simulink model "chap04_46"  (R2021a)
settings: Solver=FixedStepDiscrete  StartTime=0.0  StopTime=30  FixedStep=0.001  RelTol=1e-3
undefined symbols (not defined in the file): DiscIntNeverNeededParam
libraries: simulink x4
(part 4 of 4)

== system chap04_46/Subsystem/Subsystem2/Subsystem3/Subsystem ==
  e1 : Inport
  k3 : Inport  Port=2
  k4 : Inport  Port=3
  Add : Sum
  Constant3 : Constant  Value=-1
  Constant4 : Constant  Value=-1
  Discrete-Time Integrator1 : DiscreteIntegrator  SampleTime=-1  ICPrevOutput=DiscIntNeverNeededParam  ICPrevScaledInput=DiscIntNeverNeededParam
  Divide : Product  Inputs=*/
  MATLAB Function : MATLAB Function  TreatAsAtomicUnit=on
  Product3 : Product  Inputs=3
  Product5 : Product  Inputs=3
  z2 : Outport
  wires:
  Constant4/1 -> Product5/1
  Product5/1 -> Add/2
  Discrete-Time Integrator1/1 -> z2/1
  k3/1 -> Product3/3
  k4/1 -> Product5/3
  Divide/1 -> Add/1
  Add/1 -> Discrete-Time Integrator1/1
  Constant3/1 -> Product3/1
  e1/1 -> Product5/2, MATLAB Function/1(u), Product3/2
  MATLAB Function/1(y) -> Divide/2
  Product3/1 -> Divide/1

== system chap04_46/Subsystem/Subsystem2/Subsystem3/Subsystem1 ==
  e1 : Inport
  k1 : Inport  Port=2
  Constant : Constant  Value=-1
  Divide : Product  Inputs=*/
  MATLAB Function : MATLAB Function  TreatAsAtomicUnit=on
  Product : Product  Inputs=3
  Out1 : Outport
  wires:
  e1/1 -> Product/2, MATLAB Function/1(u)
  Divide/1 -> Out1/1
  Constant/1 -> Product/1
  k1/1 -> Product/3
  MATLAB Function/1(y) -> Divide/2
  Product/1 -> Divide/1

== system chap04_46/Subsystem/Subsystem2/Subsystem3/Subsystem2 ==
  e1 : Inport
  Constant1 : Constant  Value=0.2
  Discrete-Time Integrator1 : DiscreteIntegrator  gainval=1  InitialCondition=0.25  SampleTime=-1  ICPrevOutput=DiscIntNeverNeededParam  ICPrevScaledInput=DiscIntNeverNeededParam
  MATLAB Function : MATLAB Function  TreatAsAtomicUnit=on
  Product{,1..3,6} (5 alike) : Product
  Scope1 : Scope
  Sqrt : Sqrt  SaturateOnIntegerOverflow=on
  Square : Math  Operator=square  SaturateOnIntegerOverflow=on
  Subtract2 : Sum  Inputs=+-
  c1 : Constant  Value=0.3
  c2 : Constant  Value=0.3
  c3 : Constant  Value=0.5
  c4 : Constant  Value=0.5
  k1 : Outport
  k2 : Outport  Port=2
  k3 : Outport  Port=3
  k4 : Outport  Port=4
  wires:
  c2/1 -> Product/1
  Product/1 -> k2/1
  c3/1 -> Product1/1
  Product1/1 -> k3/1
  c4/1 -> Product2/1
  Product2/1 -> k4/1
  c1/1 -> Product3/1
  Product3/1 -> k1/1
  Sqrt/1 -> Product3/2
  Square/1 -> Product2/2
  e1/1 -> MATLAB Function/1(u)
  Product6/1 -> Subtract2/2
  MATLAB Function/1(y) -> Subtract2/1
  Subtract2/1 -> Discrete-Time Integrator1/1
  Constant1/1 -> Product6/1
  Discrete-Time Integrator1/1 -> Product6/2, Sqrt/1, Product/2, Square/1, Product1/2, Scope1/1

== system chap04_46/Subsystem/Subsystem2/Subsystem3/Subsystem3 ==
  e1 : Inport
  k2 : Inport  Port=2
  Constant2 : Constant  Value=-1
  Product2 : Product  Inputs=3
  Out1 : Outport
  wires:
  Product2/1 -> Out1/1
  e1/1 -> Product2/2
  k2/1 -> Product2/3
  Constant2/1 -> Product2/1

== system chap04_46/Subsystem/Subsystem2/Subsystem4/Subsystem ==
  zt3 : Inport
  Constant4 : Constant  Value=0
  Discrete-Time Integrator : DiscreteIntegrator  SampleTime=-1  UpperSaturationLimit=100  LowerSaturationLimit=-100  ICPrevOutput=DiscIntNeverNeededParam  ICPrevScaledInput=DiscIntNeverNeededParam
  Logical Operator : Logic  AllPortsSameDT=off  OutDataTypeStr=boolean
  MATLAB Function : MATLAB Function  TreatAsAtomicUnit=on
  Relational Operator : RelationalOperator  Operator===  OutDataTypeStr=boolean  RndMeth=Simplest
  Saturation : Saturate  UpperLimit=5  LowerLimit=-5
  Sign : Signum
  Sign1 : Signum
  Switch : Switch  Criteria=u2 > Threshold
  Out1 : Outport
  wires:
  MATLAB Function/1(y) -> Logical Operator/1
  Relational Operator/1 -> Logical Operator/2
  Constant4/1 -> Switch/1
  Sign1/1 -> Relational Operator/1
  zt3/1 -> Sign1/1, Switch/3
  Saturation/1 -> Out1/1, MATLAB Function/2(u2)
  Discrete-Time Integrator/1 -> Saturation/1, MATLAB Function/1(u1), Sign/1
  Sign/1 -> Relational Operator/2
  Logical Operator/1 -> Switch/2
  Switch/1 -> Discrete-Time Integrator/1

== system chap04_46/Subsystem/Subsystem2/Subsystem7/Subsystem ==
  zt3 : Inport
  Constant4 : Constant  Value=0
  Discrete-Time Integrator : DiscreteIntegrator  SampleTime=-1  UpperSaturationLimit=100  LowerSaturationLimit=-100  ICPrevOutput=DiscIntNeverNeededParam  ICPrevScaledInput=DiscIntNeverNeededParam
  Logical Operator : Logic  AllPortsSameDT=off  OutDataTypeStr=boolean
  MATLAB Function : MATLAB Function  TreatAsAtomicUnit=on
  Relational Operator : RelationalOperator  Operator===  OutDataTypeStr=boolean  RndMeth=Simplest
  Saturation : Saturate  UpperLimit=5  LowerLimit=-5
  Sign : Signum
  Sign1 : Signum
  Switch : Switch  Criteria=u2 > Threshold
  Out1 : Outport
  wires:
  Switch/1 -> Discrete-Time Integrator/1
  Logical Operator/1 -> Switch/2
  Sign/1 -> Relational Operator/2
  Discrete-Time Integrator/1 -> Sign/1, MATLAB Function/1(u1), Saturation/1
  Saturation/1 -> MATLAB Function/2(u2), Out1/1
  zt3/1 -> Switch/3, Sign1/1
  Sign1/1 -> Relational Operator/1
  Constant4/1 -> Switch/1
  Relational Operator/1 -> Logical Operator/2
  MATLAB Function/1(y) -> Logical Operator/1

== system chap04_46/Subsystem/Subsystem2/Subsystem8/Subsystem ==
  zt3 : Inport
  Constant4 : Constant  Value=0
  Discrete-Time Integrator : DiscreteIntegrator  SampleTime=-1  UpperSaturationLimit=100  LowerSaturationLimit=-100  ICPrevOutput=DiscIntNeverNeededParam  ICPrevScaledInput=DiscIntNeverNeededParam
  Logical Operator : Logic  AllPortsSameDT=off  OutDataTypeStr=boolean
  MATLAB Function : MATLAB Function  TreatAsAtomicUnit=on
  Relational Operator : RelationalOperator  Operator===  OutDataTypeStr=boolean  RndMeth=Simplest
  Saturation : Saturate  UpperLimit=5  LowerLimit=-5
  Sign : Signum
  Sign1 : Signum
  Switch : Switch  Criteria=u2 > Threshold
  Out1 : Outport
  wires:
  MATLAB Function/1(y) -> Logical Operator/1
  Relational Operator/1 -> Logical Operator/2
  Constant4/1 -> Switch/1
  Sign1/1 -> Relational Operator/1
  zt3/1 -> Sign1/1, Switch/3
  Saturation/1 -> Out1/1, MATLAB Function/2(u2)
  Discrete-Time Integrator/1 -> Saturation/1, MATLAB Function/1(u1), Sign/1
  Sign/1 -> Relational Operator/2
  Logical Operator/1 -> Switch/2
  Switch/1 -> Discrete-Time Integrator/1

== system chap04_46/Subsystem/Subsystem3/Subsystem3/Subsystem ==
  e1 : Inport
  k3 : Inport  Port=2
  k4 : Inport  Port=3
  Add : Sum
  Constant3 : Constant  Value=-1
  Constant4 : Constant  Value=-1
  Discrete-Time Integrator1 : DiscreteIntegrator  SampleTime=-1  ICPrevOutput=DiscIntNeverNeededParam  ICPrevScaledInput=DiscIntNeverNeededParam
  Divide : Product  Inputs=*/
  MATLAB Function : MATLAB Function  TreatAsAtomicUnit=on
  Product3 : Product  Inputs=3
  Product5 : Product  Inputs=3
  z2 : Outport
  wires:
  Constant4/1 -> Product5/1
  Product5/1 -> Add/2
  Discrete-Time Integrator1/1 -> z2/1
  k3/1 -> Product3/3
  k4/1 -> Product5/3
  Divide/1 -> Add/1
  Add/1 -> Discrete-Time Integrator1/1
  Constant3/1 -> Product3/1
  e1/1 -> Product5/2, MATLAB Function/1(u), Product3/2
  MATLAB Function/1(y) -> Divide/2
  Product3/1 -> Divide/1

== system chap04_46/Subsystem/Subsystem3/Subsystem3/Subsystem1 ==
  e1 : Inport
  k1 : Inport  Port=2
  Constant : Constant  Value=-1
  Divide : Product  Inputs=*/
  MATLAB Function : MATLAB Function  TreatAsAtomicUnit=on
  Product : Product  Inputs=3
  Out1 : Outport
  wires:
  e1/1 -> Product/2, MATLAB Function/1(u)
  Divide/1 -> Out1/1
  Constant/1 -> Product/1
  k1/1 -> Product/3
  MATLAB Function/1(y) -> Divide/2
  Product/1 -> Divide/1

== system chap04_46/Subsystem/Subsystem3/Subsystem3/Subsystem2 ==
  e1 : Inport
  Constant1 : Constant  Value=0.2
  Discrete-Time Integrator1 : DiscreteIntegrator  gainval=1  InitialCondition=0.25  SampleTime=-1  ICPrevOutput=DiscIntNeverNeededParam  ICPrevScaledInput=DiscIntNeverNeededParam
  MATLAB Function : MATLAB Function  TreatAsAtomicUnit=on
  Product{,1..3,6} (5 alike) : Product
  Scope1 : Scope
  Sqrt : Sqrt  SaturateOnIntegerOverflow=on
  Square : Math  Operator=square  SaturateOnIntegerOverflow=on
  Subtract2 : Sum  Inputs=+-
  c1 : Constant  Value=0.3
  c2 : Constant  Value=0.3
  c3 : Constant  Value=0.5
  c4 : Constant  Value=0.5
  k1 : Outport
  k2 : Outport  Port=2
  k3 : Outport  Port=3
  k4 : Outport  Port=4
  wires:
  c2/1 -> Product/1
  Product/1 -> k2/1
  c3/1 -> Product1/1
  Product1/1 -> k3/1
  c4/1 -> Product2/1
  Product2/1 -> k4/1
  c1/1 -> Product3/1
  Product3/1 -> k1/1
  Sqrt/1 -> Product3/2
  Square/1 -> Product2/2
  e1/1 -> MATLAB Function/1(u)
  Product6/1 -> Subtract2/2
  MATLAB Function/1(y) -> Subtract2/1
  Subtract2/1 -> Discrete-Time Integrator1/1
  Constant1/1 -> Product6/1
  Discrete-Time Integrator1/1 -> Product6/2, Sqrt/1, Product/2, Square/1, Product1/2, Scope1/1

== system chap04_46/Subsystem/Subsystem3/Subsystem3/Subsystem3 ==
  e1 : Inport
  k2 : Inport  Port=2
  Constant2 : Constant  Value=-1
  Product2 : Product  Inputs=3
  Out1 : Outport
  wires:
  Product2/1 -> Out1/1
  e1/1 -> Product2/2
  k2/1 -> Product2/3
  Constant2/1 -> Product2/1

== system chap04_46/Subsystem/Subsystem3/Subsystem4/Subsystem ==
  zt3 : Inport
  Constant4 : Constant  Value=0
  Discrete-Time Integrator : DiscreteIntegrator  SampleTime=-1  UpperSaturationLimit=100  LowerSaturationLimit=-100  ICPrevOutput=DiscIntNeverNeededParam  ICPrevScaledInput=DiscIntNeverNeededParam
  Logical Operator : Logic  AllPortsSameDT=off  OutDataTypeStr=boolean
  MATLAB Function : MATLAB Function  TreatAsAtomicUnit=on
  Relational Operator : RelationalOperator  Operator===  OutDataTypeStr=boolean  RndMeth=Simplest
  Saturation : Saturate  UpperLimit=5  LowerLimit=-5
  Sign : Signum
  Sign1 : Signum
  Switch : Switch  Criteria=u2 > Threshold
  Out1 : Outport
  wires:
  MATLAB Function/1(y) -> Logical Operator/1
  Relational Operator/1 -> Logical Operator/2
  Constant4/1 -> Switch/1
  Sign1/1 -> Relational Operator/1
  zt3/1 -> Sign1/1, Switch/3
  Saturation/1 -> Out1/1, MATLAB Function/2(u2)
  Discrete-Time Integrator/1 -> Saturation/1, MATLAB Function/1(u1), Sign/1
  Sign/1 -> Relational Operator/2
  Logical Operator/1 -> Switch/2
  Switch/1 -> Discrete-Time Integrator/1

== system chap04_46/Subsystem/Subsystem3/Subsystem7/Subsystem ==
  zt3 : Inport
  Constant4 : Constant  Value=0
  Discrete-Time Integrator : DiscreteIntegrator  SampleTime=-1  UpperSaturationLimit=100  LowerSaturationLimit=-100  ICPrevOutput=DiscIntNeverNeededParam  ICPrevScaledInput=DiscIntNeverNeededParam
  Logical Operator : Logic  AllPortsSameDT=off  OutDataTypeStr=boolean
  MATLAB Function : MATLAB Function  TreatAsAtomicUnit=on
  Relational Operator : RelationalOperator  Operator===  OutDataTypeStr=boolean  RndMeth=Simplest
  Saturation : Saturate  UpperLimit=5  LowerLimit=-5
  Sign : Signum
  Sign1 : Signum
  Switch : Switch  Criteria=u2 > Threshold
  Out1 : Outport
  wires:
  Switch/1 -> Discrete-Time Integrator/1
  Logical Operator/1 -> Switch/2
  Sign/1 -> Relational Operator/2
  Discrete-Time Integrator/1 -> Sign/1, MATLAB Function/1(u1), Saturation/1
  Saturation/1 -> MATLAB Function/2(u2), Out1/1
  zt3/1 -> Switch/3, Sign1/1
  Sign1/1 -> Relational Operator/1
  Constant4/1 -> Switch/1
  Relational Operator/1 -> Logical Operator/2
  MATLAB Function/1(y) -> Logical Operator/1

== system chap04_46/Subsystem/Subsystem3/Subsystem8/Subsystem ==
  zt3 : Inport
  Constant4 : Constant  Value=0
  Discrete-Time Integrator : DiscreteIntegrator  SampleTime=-1  UpperSaturationLimit=100  LowerSaturationLimit=-100  ICPrevOutput=DiscIntNeverNeededParam  ICPrevScaledInput=DiscIntNeverNeededParam
  Logical Operator : Logic  AllPortsSameDT=off  OutDataTypeStr=boolean
  MATLAB Function : MATLAB Function  TreatAsAtomicUnit=on
  Relational Operator : RelationalOperator  Operator===  OutDataTypeStr=boolean  RndMeth=Simplest
  Saturation : Saturate  UpperLimit=5  LowerLimit=-5
  Sign : Signum
  Sign1 : Signum
  Switch : Switch  Criteria=u2 > Threshold
  Out1 : Outport
  wires:
  MATLAB Function/1(y) -> Logical Operator/1
  Relational Operator/1 -> Logical Operator/2
  Constant4/1 -> Switch/1
  Sign1/1 -> Relational Operator/1
  zt3/1 -> Sign1/1, Switch/3
  Saturation/1 -> Out1/1, MATLAB Function/2(u2)
  Discrete-Time Integrator/1 -> Saturation/1, MATLAB Function/1(u1), Sign/1
  Sign/1 -> Relational Operator/2
  Logical Operator/1 -> Switch/2
  Switch/1 -> Discrete-Time Integrator/1

== system chap04_46/Subsystem/Subsystem4/Subsystem3/Subsystem ==
  e1 : Inport
  k3 : Inport  Port=2
  k4 : Inport  Port=3
  Add : Sum
  Constant3 : Constant  Value=-1
  Constant4 : Constant  Value=-1
  Discrete-Time Integrator1 : DiscreteIntegrator  SampleTime=-1  ICPrevOutput=DiscIntNeverNeededParam  ICPrevScaledInput=DiscIntNeverNeededParam
  Divide : Product  Inputs=*/
  MATLAB Function : MATLAB Function  TreatAsAtomicUnit=on
  Product3 : Product  Inputs=3
  Product5 : Product  Inputs=3
  z2 : Outport
  wires:
  Constant4/1 -> Product5/1
  Product5/1 -> Add/2
  Discrete-Time Integrator1/1 -> z2/1
  k3/1 -> Product3/3
  k4/1 -> Product5/3
  Divide/1 -> Add/1
  Add/1 -> Discrete-Time Integrator1/1
  Constant3/1 -> Product3/1
  e1/1 -> Product5/2, MATLAB Function/1(u), Product3/2
  MATLAB Function/1(y) -> Divide/2
  Product3/1 -> Divide/1

== system chap04_46/Subsystem/Subsystem4/Subsystem3/Subsystem1 ==
  e1 : Inport
  k1 : Inport  Port=2
  Constant : Constant  Value=-1
  Divide : Product  Inputs=*/
  MATLAB Function : MATLAB Function  TreatAsAtomicUnit=on
  Product : Product  Inputs=3
  Out1 : Outport
  wires:
  e1/1 -> Product/2, MATLAB Function/1(u)
  Divide/1 -> Out1/1
  Constant/1 -> Product/1
  k1/1 -> Product/3
  MATLAB Function/1(y) -> Divide/2
  Product/1 -> Divide/1

== system chap04_46/Subsystem/Subsystem4/Subsystem3/Subsystem2 ==
  e1 : Inport
  Constant1 : Constant  Value=0.2
  Discrete-Time Integrator1 : DiscreteIntegrator  gainval=1  InitialCondition=0.25  SampleTime=-1  ICPrevOutput=DiscIntNeverNeededParam  ICPrevScaledInput=DiscIntNeverNeededParam
  MATLAB Function : MATLAB Function  TreatAsAtomicUnit=on
  Product{,1..3,6} (5 alike) : Product
  Scope1 : Scope
  Sqrt : Sqrt  SaturateOnIntegerOverflow=on
  Square : Math  Operator=square  SaturateOnIntegerOverflow=on
  Subtract2 : Sum  Inputs=+-
  c1 : Constant  Value=0.3
  c2 : Constant  Value=0.3
  c3 : Constant  Value=0.5
  c4 : Constant  Value=0.5
  k1 : Outport
  k2 : Outport  Port=2
  k3 : Outport  Port=3
  k4 : Outport  Port=4
  wires:
  c2/1 -> Product/1
  Product/1 -> k2/1
  c3/1 -> Product1/1
  Product1/1 -> k3/1
  c4/1 -> Product2/1
  Product2/1 -> k4/1
  c1/1 -> Product3/1
  Product3/1 -> k1/1
  Sqrt/1 -> Product3/2
  Square/1 -> Product2/2
  e1/1 -> MATLAB Function/1(u)
  Product6/1 -> Subtract2/2
  MATLAB Function/1(y) -> Subtract2/1
  Subtract2/1 -> Discrete-Time Integrator1/1
  Constant1/1 -> Product6/1
  Discrete-Time Integrator1/1 -> Product6/2, Sqrt/1, Product/2, Square/1, Product1/2, Scope1/1

== system chap04_46/Subsystem/Subsystem4/Subsystem3/Subsystem3 ==
  e1 : Inport
  k2 : Inport  Port=2
  Constant2 : Constant  Value=-1
  Product2 : Product  Inputs=3
  Out1 : Outport
  wires:
  Product2/1 -> Out1/1
  e1/1 -> Product2/2
  k2/1 -> Product2/3
  Constant2/1 -> Product2/1

== system chap04_46/Subsystem/Subsystem4/Subsystem4/Subsystem ==
  zt3 : Inport
  Constant4 : Constant  Value=0
  Discrete-Time Integrator : DiscreteIntegrator  SampleTime=-1  UpperSaturationLimit=100  LowerSaturationLimit=-100  ICPrevOutput=DiscIntNeverNeededParam  ICPrevScaledInput=DiscIntNeverNeededParam
  Logical Operator : Logic  AllPortsSameDT=off  OutDataTypeStr=boolean
  MATLAB Function : MATLAB Function  TreatAsAtomicUnit=on
  Relational Operator : RelationalOperator  Operator===  OutDataTypeStr=boolean  RndMeth=Simplest
  Saturation : Saturate  UpperLimit=5  LowerLimit=-5
  Sign : Signum
  Sign1 : Signum
  Switch : Switch  Criteria=u2 > Threshold
  Out1 : Outport
  wires:
  MATLAB Function/1(y) -> Logical Operator/1
  Relational Operator/1 -> Logical Operator/2
  Constant4/1 -> Switch/1
  Sign1/1 -> Relational Operator/1
  zt3/1 -> Sign1/1, Switch/3
  Saturation/1 -> Out1/1, MATLAB Function/2(u2)
  Discrete-Time Integrator/1 -> Saturation/1, MATLAB Function/1(u1), Sign/1
  Sign/1 -> Relational Operator/2
  Logical Operator/1 -> Switch/2
  Switch/1 -> Discrete-Time Integrator/1

== system chap04_46/Subsystem/Subsystem4/Subsystem7/Subsystem ==
  zt3 : Inport
  Constant4 : Constant  Value=0
  Discrete-Time Integrator : DiscreteIntegrator  SampleTime=-1  UpperSaturationLimit=100  LowerSaturationLimit=-100  ICPrevOutput=DiscIntNeverNeededParam  ICPrevScaledInput=DiscIntNeverNeededParam
  Logical Operator : Logic  AllPortsSameDT=off  OutDataTypeStr=boolean
  MATLAB Function : MATLAB Function  TreatAsAtomicUnit=on
  Relational Operator : RelationalOperator  Operator===  OutDataTypeStr=boolean  RndMeth=Simplest
  Saturation : Saturate  UpperLimit=5  LowerLimit=-5
  Sign : Signum
  Sign1 : Signum
  Switch : Switch  Criteria=u2 > Threshold
  Out1 : Outport
  wires:
  Switch/1 -> Discrete-Time Integrator/1
  Logical Operator/1 -> Switch/2
  Sign/1 -> Relational Operator/2
  Discrete-Time Integrator/1 -> Sign/1, MATLAB Function/1(u1), Saturation/1
  Saturation/1 -> MATLAB Function/2(u2), Out1/1
  zt3/1 -> Switch/3, Sign1/1
  Sign1/1 -> Relational Operator/1
  Constant4/1 -> Switch/1
  Relational Operator/1 -> Logical Operator/2
  MATLAB Function/1(y) -> Logical Operator/1

== system chap04_46/Subsystem/Subsystem4/Subsystem8/Subsystem ==
  zt3 : Inport
  Constant4 : Constant  Value=0
  Discrete-Time Integrator : DiscreteIntegrator  SampleTime=-1  UpperSaturationLimit=100  LowerSaturationLimit=-100  ICPrevOutput=DiscIntNeverNeededParam  ICPrevScaledInput=DiscIntNeverNeededParam
  Logical Operator : Logic  AllPortsSameDT=off  OutDataTypeStr=boolean
  MATLAB Function : MATLAB Function  TreatAsAtomicUnit=on
  Relational Operator : RelationalOperator  Operator===  OutDataTypeStr=boolean  RndMeth=Simplest
  Saturation : Saturate  UpperLimit=5  LowerLimit=-5
  Sign : Signum
  Sign1 : Signum
  Switch : Switch  Criteria=u2 > Threshold
  Out1 : Outport
  wires:
  MATLAB Function/1(y) -> Logical Operator/1
  Relational Operator/1 -> Logical Operator/2
  Constant4/1 -> Switch/1
  Sign1/1 -> Relational Operator/1
  zt3/1 -> Sign1/1, Switch/3
  Saturation/1 -> Out1/1, MATLAB Function/2(u2)
  Discrete-Time Integrator/1 -> Saturation/1, MATLAB Function/1(u1), Sign/1
  Sign/1 -> Relational Operator/2
  Logical Operator/1 -> Switch/2
  Switch/1 -> Discrete-Time Integrator/1

== system chap04_46/Subsystem/Subsystem5/Subsystem3/Subsystem ==
  e1 : Inport
  k3 : Inport  Port=2
  k4 : Inport  Port=3
  Add : Sum
  Constant3 : Constant  Value=-1
  Constant4 : Constant  Value=-1
  Discrete-Time Integrator1 : DiscreteIntegrator  SampleTime=-1  ICPrevOutput=DiscIntNeverNeededParam  ICPrevScaledInput=DiscIntNeverNeededParam
  Divide : Product  Inputs=*/
  MATLAB Function : MATLAB Function  TreatAsAtomicUnit=on
  Product3 : Product  Inputs=3
  Product5 : Product  Inputs=3
  z2 : Outport
  wires:
  Constant4/1 -> Product5/1
  Product5/1 -> Add/2
  Discrete-Time Integrator1/1 -> z2/1
  k3/1 -> Product3/3
  k4/1 -> Product5/3
  Divide/1 -> Add/1
  Add/1 -> Discrete-Time Integrator1/1
  Constant3/1 -> Product3/1
  e1/1 -> Product5/2, MATLAB Function/1(u), Product3/2
  MATLAB Function/1(y) -> Divide/2
  Product3/1 -> Divide/1

== system chap04_46/Subsystem/Subsystem5/Subsystem3/Subsystem1 ==
  e1 : Inport
  k1 : Inport  Port=2
  Constant : Constant  Value=-1
  Divide : Product  Inputs=*/
  MATLAB Function : MATLAB Function  TreatAsAtomicUnit=on
  Product : Product  Inputs=3
  Out1 : Outport
  wires:
  e1/1 -> Product/2, MATLAB Function/1(u)
  Divide/1 -> Out1/1
  Constant/1 -> Product/1
  k1/1 -> Product/3
  MATLAB Function/1(y) -> Divide/2
  Product/1 -> Divide/1

== system chap04_46/Subsystem/Subsystem5/Subsystem3/Subsystem2 ==
  e1 : Inport
  Constant1 : Constant  Value=0.2
  Discrete-Time Integrator1 : DiscreteIntegrator  gainval=1  InitialCondition=0.25  SampleTime=-1  ICPrevOutput=DiscIntNeverNeededParam  ICPrevScaledInput=DiscIntNeverNeededParam
  MATLAB Function : MATLAB Function  TreatAsAtomicUnit=on
  Product{,1..3,6} (5 alike) : Product
  Scope1 : Scope
  Sqrt : Sqrt  SaturateOnIntegerOverflow=on
  Square : Math  Operator=square  SaturateOnIntegerOverflow=on
  Subtract2 : Sum  Inputs=+-
  c1 : Constant  Value=0.3
  c2 : Constant  Value=0.3
  c3 : Constant  Value=0.5
  c4 : Constant  Value=0.5
  k1 : Outport
  k2 : Outport  Port=2
  k3 : Outport  Port=3
  k4 : Outport  Port=4
  wires:
  c2/1 -> Product/1
  Product/1 -> k2/1
  c3/1 -> Product1/1
  Product1/1 -> k3/1
  c4/1 -> Product2/1
  Product2/1 -> k4/1
  c1/1 -> Product3/1
  Product3/1 -> k1/1
  Sqrt/1 -> Product3/2
  Square/1 -> Product2/2
  e1/1 -> MATLAB Function/1(u)
  Product6/1 -> Subtract2/2
  MATLAB Function/1(y) -> Subtract2/1
  Subtract2/1 -> Discrete-Time Integrator1/1
  Constant1/1 -> Product6/1
  Discrete-Time Integrator1/1 -> Product6/2, Sqrt/1, Product/2, Square/1, Product1/2, Scope1/1

== system chap04_46/Subsystem/Subsystem5/Subsystem3/Subsystem3 ==
  e1 : Inport
  k2 : Inport  Port=2
  Constant2 : Constant  Value=-1
  Product2 : Product  Inputs=3
  Out1 : Outport
  wires:
  Product2/1 -> Out1/1
  e1/1 -> Product2/2
  k2/1 -> Product2/3
  Constant2/1 -> Product2/1

== system chap04_46/Subsystem/Subsystem5/Subsystem4/Subsystem ==
  zt3 : Inport
  Constant4 : Constant  Value=0
  Discrete-Time Integrator : DiscreteIntegrator  SampleTime=-1  UpperSaturationLimit=100  LowerSaturationLimit=-100  ICPrevOutput=DiscIntNeverNeededParam  ICPrevScaledInput=DiscIntNeverNeededParam
  Logical Operator : Logic  AllPortsSameDT=off  OutDataTypeStr=boolean
  MATLAB Function : MATLAB Function  TreatAsAtomicUnit=on
  Relational Operator : RelationalOperator  Operator===  OutDataTypeStr=boolean  RndMeth=Simplest
  Saturation : Saturate  UpperLimit=5  LowerLimit=-5
  Sign : Signum
  Sign1 : Signum
  Switch : Switch  Criteria=u2 > Threshold
  Out1 : Outport
  wires:
  MATLAB Function/1(y) -> Logical Operator/1
  Relational Operator/1 -> Logical Operator/2
  Constant4/1 -> Switch/1
  Sign1/1 -> Relational Operator/1
  zt3/1 -> Sign1/1, Switch/3
  Saturation/1 -> Out1/1, MATLAB Function/2(u2)
  Discrete-Time Integrator/1 -> Saturation/1, MATLAB Function/1(u1), Sign/1
  Sign/1 -> Relational Operator/2
  Logical Operator/1 -> Switch/2
  Switch/1 -> Discrete-Time Integrator/1

== system chap04_46/Subsystem/Subsystem5/Subsystem7/Subsystem ==
  zt3 : Inport
  Constant4 : Constant  Value=0
  Discrete-Time Integrator : DiscreteIntegrator  SampleTime=-1  UpperSaturationLimit=100  LowerSaturationLimit=-100  ICPrevOutput=DiscIntNeverNeededParam  ICPrevScaledInput=DiscIntNeverNeededParam
  Logical Operator : Logic  AllPortsSameDT=off  OutDataTypeStr=boolean
  MATLAB Function : MATLAB Function  TreatAsAtomicUnit=on
  Relational Operator : RelationalOperator  Operator===  OutDataTypeStr=boolean  RndMeth=Simplest
  Saturation : Saturate  UpperLimit=5  LowerLimit=-5
  Sign : Signum
  Sign1 : Signum
  Switch : Switch  Criteria=u2 > Threshold
  Out1 : Outport
  wires:
  Switch/1 -> Discrete-Time Integrator/1
  Logical Operator/1 -> Switch/2
  Sign/1 -> Relational Operator/2
  Discrete-Time Integrator/1 -> Sign/1, MATLAB Function/1(u1), Saturation/1
  Saturation/1 -> MATLAB Function/2(u2), Out1/1
  zt3/1 -> Switch/3, Sign1/1
  Sign1/1 -> Relational Operator/1
  Constant4/1 -> Switch/1
  Relational Operator/1 -> Logical Operator/2
  MATLAB Function/1(y) -> Logical Operator/1

== system chap04_46/Subsystem/Subsystem5/Subsystem8/Subsystem ==
  zt3 : Inport
  Constant4 : Constant  Value=0
  Discrete-Time Integrator : DiscreteIntegrator  SampleTime=-1  UpperSaturationLimit=100  LowerSaturationLimit=-100  ICPrevOutput=DiscIntNeverNeededParam  ICPrevScaledInput=DiscIntNeverNeededParam
  Logical Operator : Logic  AllPortsSameDT=off  OutDataTypeStr=boolean
  MATLAB Function : MATLAB Function  TreatAsAtomicUnit=on
  Relational Operator : RelationalOperator  Operator===  OutDataTypeStr=boolean  RndMeth=Simplest
  Saturation : Saturate  UpperLimit=5  LowerLimit=-5
  Sign : Signum
  Sign1 : Signum
  Switch : Switch  Criteria=u2 > Threshold
  Out1 : Outport
  wires:
  MATLAB Function/1(y) -> Logical Operator/1
  Relational Operator/1 -> Logical Operator/2
  Constant4/1 -> Switch/1
  Sign1/1 -> Relational Operator/1
  zt3/1 -> Sign1/1, Switch/3
  Saturation/1 -> Out1/1, MATLAB Function/2(u2)
  Discrete-Time Integrator/1 -> Saturation/1, MATLAB Function/1(u1), Sign/1
  Sign/1 -> Relational Operator/2
  Logical Operator/1 -> Switch/2
  Switch/1 -> Discrete-Time Integrator/1

== matlab function chap04_46/Subsystem/Subsystem/Subsystem4/Subsystem/MATLAB Function ==
  data: u1 input; y output; u2 input
function y = fcn(u1,u2)


if (u1==u2)
    y = 0;
else
    y = 1;
end

== matlab function chap04_46/Subsystem/Subsystem5/Subsystem12/MATLAB Function ==
  data: u input; y output
function y = fcn(u)

y = norm(u);

== matlab function chap04_46/Subsystem/Subsystem5/Subsystem4/Subsystem/MATLAB Function ==
  data: u1 input; y output; u2 input
function y = fcn(u1,u2)


if (u1==u2)
    y = 0;
else
    y = 1;
end

== matlab function chap04_46/Subsystem/Subsystem5/Subsystem7/Subsystem/MATLAB Function ==
  data: u1 input; y output; u2 input
function y = fcn(u1,u2)


if (u1==u2)
    y = 0;
else
    y = 1;
end

== matlab function chap04_46/Subsystem/Subsystem5/Subsystem8/Subsystem/MATLAB Function ==
  data: u1 input; y output; u2 input
function y = fcn(u1,u2)


if (u1==u2)
    y = 0;
else
    y = 1;
end

== matlab function chap04_46/Subsystem/Subsystem5/Subsystem12/MATLAB Function3 ==
  data: u input; y output
function y = fcn(u)

y = norm(u);

== matlab function chap04_46/Subsystem/Subsystem3/Subsystem12/MATLAB Function ==
  data: u input; y output
function y = fcn(u)

y = norm(u);

== matlab function chap04_46/Subsystem/Subsystem3/Subsystem12/MATLAB Function3 ==
  data: u input; y output
function y = fcn(u)

y = norm(u);

== matlab function chap04_46/Subsystem/Subsystem2/Subsystem7/Subsystem/MATLAB Function ==
  data: u1 input; y output; u2 input
function y = fcn(u1,u2)


if (u1==u2)
    y = 0;
else
    y = 1;
end

== matlab function chap04_46/Subsystem/Subsystem3/Subsystem4/Subsystem/MATLAB Function ==
  data: u1 input; y output; u2 input
function y = fcn(u1,u2)


if (u1==u2)
    y = 0;
else
    y = 1;
end

== matlab function chap04_46/Subsystem/Subsystem3/Subsystem7/Subsystem/MATLAB Function ==
  data: u1 input; y output; u2 input
function y = fcn(u1,u2)


if (u1==u2)
    y = 0;
else
    y = 1;
end

== matlab function chap04_46/Subsystem/Subsystem4/Subsystem4/Subsystem/MATLAB Function ==
  data: u1 input; y output; u2 input
function y = fcn(u1,u2)


if (u1==u2)
    y = 0;
else
    y = 1;
end

== matlab function chap04_46/Subsystem/Subsystem4/Subsystem7/Subsystem/MATLAB Function ==
  data: u1 input; y output; u2 input
function y = fcn(u1,u2)


if (u1==u2)
    y = 0;
else
    y = 1;
end

== matlab function chap04_46/Subsystem/Subsystem4/Subsystem8/Subsystem/MATLAB Function ==
  data: u1 input; y output; u2 input
function y = fcn(u1,u2)


if (u1==u2)
    y = 0;
else
    y = 1;
end

== matlab function chap04_46/Subsystem/Subsystem3/Subsystem8/Subsystem/MATLAB Function ==
  data: u1 input; y output; u2 input
function y = fcn(u1,u2)


if (u1==u2)
    y = 0;
else
    y = 1;
end

== matlab function chap04_46/Subsystem/Subsystem1/Subsystem12/MATLAB Function ==
  data: u input; y output
function y = fcn(u)

y = norm(u);

== matlab function chap04_46/Subsystem/Subsystem1/Subsystem12/MATLAB Function3 ==
  data: u input; y output
function y = fcn(u)

y = norm(u);

== matlab function chap04_46/Subsystem/Subsystem4/Subsystem12/MATLAB Function ==
  data: u input; y output
function y = fcn(u)

y = norm(u);

== matlab function chap04_46/Subsystem/Subsystem4/Subsystem12/MATLAB Function3 ==
  data: u input; y output
function y = fcn(u)

y = norm(u);

== matlab function chap04_46/Subsystem/Subsystem2/Subsystem3/Subsystem2/MATLAB Function ==
  data: u input; y output
function y = fcn(u)

y = norm(u);

== matlab function chap04_46/Subsystem/Subsystem2/Subsystem8/Subsystem/MATLAB Function ==
  data: u1 input; y output; u2 input
function y = fcn(u1,u2)


if (u1==u2)
    y = 0;
else
    y = 1;
end

== matlab function chap04_46/Subsystem/Subsystem5/Subsystem3/Subsystem2/MATLAB Function ==
  data: u input; y output
function y = fcn(u)

y = norm(u);

== matlab function chap04_46/Subsystem/Subsystem3/Subsystem3/Subsystem2/MATLAB Function ==
  data: u input; y output
function y = fcn(u)

y = norm(u);

== matlab function chap04_46/Subsystem/Subsystem1/Subsystem3/Subsystem2/MATLAB Function ==
  data: u input; y output
function y = fcn(u)

y = norm(u);

== matlab function chap04_46/Subsystem/Subsystem4/Subsystem3/Subsystem2/MATLAB Function ==
  data: u input; y output
function y = fcn(u)

y = norm(u);

== matlab function chap04_46/Subsystem/Subsystem/Subsystem3/MATLAB Function ==
  data: u input; y output
function y = fcn(u)

y = u;

if y==0
    y=10e-15;
end

== matlab function chap04_46/Subsystem/Subsystem/Subsystem3/MATLAB Function1 ==
  data: u input; y output
function y = fcn(u)

y = u;

if y==0
    y=10e-15;
end

== matlab function chap04_46/Subsystem/Subsystem/Subsystem3/MATLAB Function2 ==
  data: u input; y output
function y = fcn(u)

y = u;

if y==0
    y=10e-15;
end

== matlab function chap04_46/Subsystem/Subsystem/Subsystem3/Subsystem/MATLAB Function ==
  data: u input; y output
function y = fcn(u)

y = norm(u);

== matlab function chap04_46/Subsystem/Subsystem/Subsystem3/Subsystem1/MATLAB Function ==
  data: u input; y output
function y = fcn(u)

y = norm(u)^(1/2);

== matlab function chap04_46/Subsystem/Subsystem/Subsystem3/Subsystem2/MATLAB Function ==
  data: u input; y output
function y = fcn(u)

y = norm(u);

== matlab function chap04_46/Subsystem/Subsystem2/Subsystem3/MATLAB Function ==
  data: u input; y output
function y = fcn(u)

y = u;

if y==0
    y=10e-15;
end

== matlab function chap04_46/Subsystem/Subsystem1/Subsystem4/Subsystem/MATLAB Function ==
  data: u1 input; y output; u2 input
function y = fcn(u1,u2)


if (u1==u2)
    y = 0;
else
    y = 1;
end

== matlab function chap04_46/Subsystem/Subsystem2/Subsystem3/MATLAB Function1 ==
  data: u input; y output
function y = fcn(u)

y = u;

if y==0
    y=10e-15;
end

== matlab function chap04_46/Subsystem/Subsystem2/Subsystem3/MATLAB Function2 ==
  data: u input; y output
function y = fcn(u)

y = u;

if y==0
    y=10e-15;
end

== matlab function chap04_46/Subsystem/Subsystem2/Subsystem3/Subsystem/MATLAB Function ==
  data: u input; y output
function y = fcn(u)

y = norm(u);

== matlab function chap04_46/Subsystem/Subsystem2/Subsystem3/Subsystem1/MATLAB Function ==
  data: u input; y output
function y = fcn(u)

y = norm(u)^(1/2);

== matlab function chap04_46/Subsystem/Subsystem5/Subsystem3/MATLAB Function ==
  data: u input; y output
function y = fcn(u)

y = u;

if y==0
    y=10e-15;
end

== matlab function chap04_46/Subsystem/Subsystem5/Subsystem3/MATLAB Function1 ==
  data: u input; y output
function y = fcn(u)

y = u;

if y==0
    y=10e-15;
end

== matlab function chap04_46/Subsystem/Subsystem5/Subsystem3/MATLAB Function2 ==
  data: u input; y output
function y = fcn(u)

y = u;

if y==0
    y=10e-15;
end

== matlab function chap04_46/Subsystem/Subsystem5/Subsystem3/Subsystem/MATLAB Function ==
  data: u input; y output
function y = fcn(u)

y = norm(u);

== matlab function chap04_46/Subsystem/Subsystem5/Subsystem3/Subsystem1/MATLAB Function ==
  data: u input; y output
function y = fcn(u)

y = norm(u)^(1/2);

== matlab function chap04_46/Subsystem/Subsystem3/Subsystem3/MATLAB Function ==
  data: u input; y output
function y = fcn(u)

y = u;

if y==0
    y=10e-15;
end

== matlab function chap04_46/Subsystem/Subsystem3/Subsystem3/MATLAB Function1 ==
  data: u input; y output
function y = fcn(u)

y = u;

if y==0
    y=10e-15;
end

== matlab function chap04_46/Subsystem/Subsystem3/Subsystem3/MATLAB Function2 ==
  data: u input; y output
function y = fcn(u)

y = u;

if y==0
    y=10e-15;
end

== matlab function chap04_46/Subsystem/Subsystem1/Subsystem7/Subsystem/MATLAB Function ==
  data: u1 input; y output; u2 input
function y = fcn(u1,u2)


if (u1==u2)
    y = 0;
else
    y = 1;
end

== matlab function chap04_46/Subsystem/Subsystem3/Subsystem3/Subsystem/MATLAB Function ==
  data: u input; y output
function y = fcn(u)

y = norm(u);

== matlab function chap04_46/Subsystem/Subsystem3/Subsystem3/Subsystem1/MATLAB Function ==
  data: u input; y output
function y = fcn(u)

y = norm(u)^(1/2);

== matlab function chap04_46/Subsystem/Subsystem1/Subsystem3/MATLAB Function ==
  data: u input; y output
function y = fcn(u)

y = u;

if y==0
    y=10e-15;
end

== matlab function chap04_46/Subsystem/Subsystem1/Subsystem3/MATLAB Function1 ==
  data: u input; y output
function y = fcn(u)

y = u;

if y==0
    y=10e-15;
end

== matlab function chap04_46/Subsystem/Subsystem1/Subsystem3/MATLAB Function2 ==
  data: u input; y output
function y = fcn(u)

y = u;

if y==0
    y=10e-15;
end

== matlab function chap04_46/Subsystem/Subsystem1/Subsystem3/Subsystem/MATLAB Function ==
  data: u input; y output
function y = fcn(u)

y = norm(u);

== matlab function chap04_46/Subsystem/Subsystem1/Subsystem3/Subsystem1/MATLAB Function ==
  data: u input; y output
function y = fcn(u)

y = norm(u)^(1/2);

== matlab function chap04_46/Subsystem/Subsystem4/Subsystem3/MATLAB Function ==
  data: u input; y output
function y = fcn(u)

y = u;

if y==0
    y=10e-15;
end

== matlab function chap04_46/Subsystem/Subsystem4/Subsystem3/MATLAB Function1 ==
  data: u input; y output
function y = fcn(u)

y = u;

if y==0
    y=10e-15;
end

== matlab function chap04_46/Subsystem/Subsystem4/Subsystem3/MATLAB Function2 ==
  data: u input; y output
function y = fcn(u)

y = u;

if y==0
    y=10e-15;
end

== matlab function chap04_46/Subsystem/Subsystem4/Subsystem3/Subsystem/MATLAB Function ==
  data: u input; y output
function y = fcn(u)

y = norm(u);

== matlab function chap04_46/Subsystem/Subsystem1/Subsystem8/Subsystem/MATLAB Function ==
  data: u1 input; y output; u2 input
function y = fcn(u1,u2)


if (u1==u2)
    y = 0;
else
    y = 1;
end

== matlab function chap04_46/Subsystem/Subsystem4/Subsystem3/Subsystem1/MATLAB Function ==
  data: u input; y output
function y = fcn(u)

y = norm(u)^(1/2);

== matlab function chap04_46/Subsystem/Subsystem/Subsystem7/Subsystem/MATLAB Function ==
  data: u1 input; y output; u2 input
function y = fcn(u1,u2)


if (u1==u2)
    y = 0;
else
    y = 1;
end

== matlab function chap04_46/Subsystem/Subsystem/Subsystem8/Subsystem/MATLAB Function ==
  data: u1 input; y output; u2 input
function y = fcn(u1,u2)


if (u1==u2)
    y = 0;
else
    y = 1;
end

== matlab function chap04_46/Subsystem/Subsystem2/Subsystem12/MATLAB Function ==
  data: u input; y output
function y = fcn(u)

y = norm(u);

== matlab function chap04_46/Subsystem/Subsystem/Subsystem12/MATLAB Function ==
  data: u input; y output
function y = fcn(u)

y = norm(u);

== matlab function chap04_46/Subsystem/Subsystem2/Subsystem4/Subsystem/MATLAB Function ==
  data: u1 input; y output; u2 input
function y = fcn(u1,u2)


if (u1==u2)
    y = 0;
else
    y = 1;
end

== matlab function chap04_46/Subsystem/Subsystem/Subsystem12/MATLAB Function3 ==
  data: u input; y output
function y = fcn(u)

y = norm(u);

== matlab function chap04_46/Subsystem/Subsystem2/Subsystem12/MATLAB Function3 ==
  data: u input; y output
function y = fcn(u)

y = norm(u);
